simulink model "ModuladorTorqueEquivalente"  (R2023b)
settings: Solver=VariableStepAuto  StartTime=0.0  StopTime=10.0  RelTol=1e-3
values from neighbouring files (symbols this model uses):
  b_eq = b_m + b_l/(r^2)    (= 2.19444444444e-05)    [Parametros.m]
  k_l = m*l_cm + m_l(1)*l_l    [Parametros.m]
  L_d = 6.6E-3    (= 0.0066)    [Parametros.m]
  L_ls = 0.8E-3    (= 0.0008)    [Parametros.m]
  L_q = 5.8E-3    (= 0.0058)    [Parametros.m]
  lambda_m = 0.016    [Parametros.m]
  P_p = 3    [Parametros.m]
  r = 120    [MigracionPolosControladorExterno.m]    (also in Parametros.m)
settings Model: Creator=matia  LastModifiedBy=matia

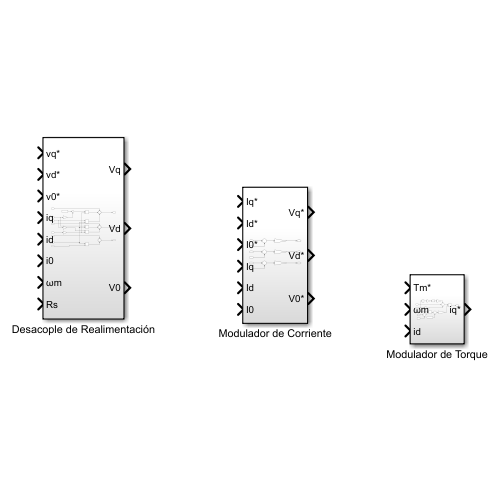
[thumbnail: Simulink's stored preview of the top-level diagram]
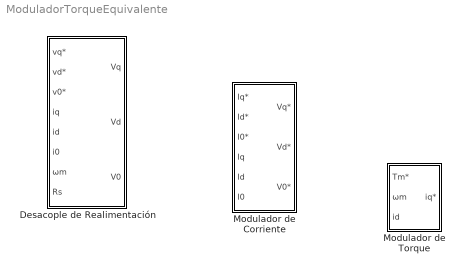
== system ModuladorTorqueEquivalente ==
  Desacople de Realimentación : Subsystem
  Modulador de Corriente : Subsystem
  Modulador de Torque : Subsystem

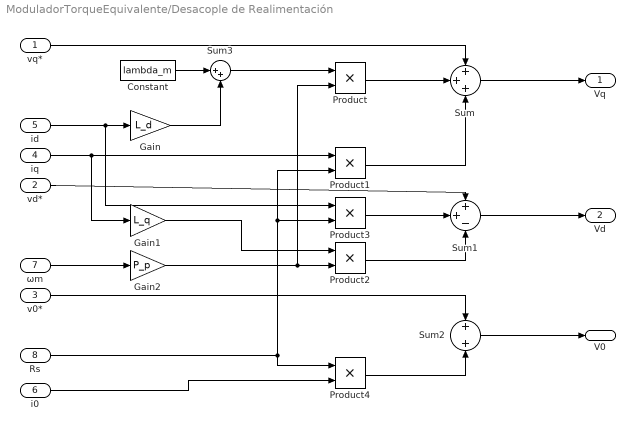
== system ModuladorTorqueEquivalente/Desacople de Realimentación ==
  vq* : Inport
  vd* : Inport  Port=2
  v0* : Inport  Port=3
  iq : Inport  Port=4
  id : Inport  Port=5
  i0 : Inport  Port=6
  ωm : Inport  Port=7
  Rs : Inport  Port=8
  Constant : Constant  Value=lambda_m
  Gain : Gain  Gain=L_d
  Gain1 : Gain  Gain=L_q
  Gain2 : Gain  Gain=P_p
  Product{,1..4} (5 alike) : Product
  Sum : Sum  Inputs=+++
  Sum1 : Sum  Inputs=++-
  Sum2 : Sum  Inputs=+|+
  Sum3 : Sum  Inputs=|++
  Vq : Outport
  Vd : Outport  Port=2
  V0 : Outport  Port=3
  wires:
  ωm/1 -> Gain2/1
  Sum/1 -> Vq/1
  Rs/1 -> Product4/1, Product1/2, Product3/2
  Gain/1 -> Sum3/2
  Product/1 -> Sum/2
  Sum2/1 -> V0/1
  Product4/1 -> Sum2/2
  Sum3/1 -> Product/1
  id/1 -> Product3/1, Gain/1
  vq*/1 -> Sum/1
  i0/1 -> Product4/2
  iq/1 -> Product1/1, Gain1/1
  Product2/1 -> Sum1/3
  Constant/1 -> Sum3/1
  v0*/1 -> Sum2/1
  Product1/1 -> Sum/3
  Gain2/1 -> Product/2, Product2/2
  vd*/1 -> Sum1/1
  Gain1/1 -> Product2/1
  Sum1/1 -> Vd/1
  Product3/1 -> Sum1/2

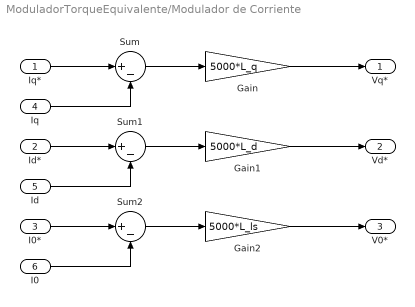
== system ModuladorTorqueEquivalente/Modulador de Corriente ==
  Iq* : Inport
  Id* : Inport  Port=2
  I0* : Inport  Port=3
  Iq : Inport  Port=4
  Id : Inport  Port=5
  I0 : Inport  Port=6
  Gain : Gain  Gain=5000*L_q
  Gain1 : Gain  Gain=5000*L_d
  Gain2 : Gain  Gain=5000*L_ls
  Sum : Sum  Inputs=|+-
  Sum1 : Sum  Inputs=|+-
  Sum2 : Sum  Inputs=|+-
  Vq* : Outport
  Vd* : Outport  Port=2
  V0* : Outport  Port=3
  wires:
  Gain2/1 -> V0*/1
  Sum/1 -> Gain/1
  Sum1/1 -> Gain1/1
  Gain/1 -> Vq*/1
  Iq/1 -> Sum/2
  I0*/1 -> Sum2/1
  Iq*/1 -> Sum/1
  Id/1 -> Sum1/2
  Sum2/1 -> Gain2/1
  Id*/1 -> Sum1/1
  Gain1/1 -> Vd*/1
  I0/1 -> Sum2/2

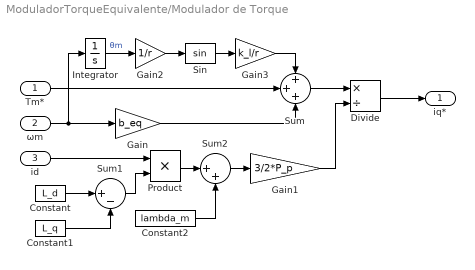
== system ModuladorTorqueEquivalente/Modulador de Torque ==
  Tm* : Inport
  ωm : Inport  Port=2
  id : Inport  Port=3
  Constant : Constant  Value=L_d
  Constant1 : Constant  Value=L_q
  Constant2 : Constant  Value=lambda_m
  Divide : Product  Inputs=*/
  Gain : Gain  Gain=b_eq
  Gain1 : Gain  Gain=3/2*P_p
  Gain2 : Gain  Gain=1/r
  Gain3 : Gain  Gain=k_l/r
  Integrator : Integrator
  Product : Product
  Sin : Trigonometry
  Sum : Sum  Inputs=+++
  Sum1 : Sum  Inputs=|+-
  Sum2 : Sum  Inputs=|++
  iq* : Outport
  wires:
  Constant2/1 -> Sum2/2
  ωm/1 -> Gain/1, Integrator/1
  Sum1/1 -> Product/2
  Gain3/1 -> Sum/1
  Integrator/1 -> Gain2/1  "θm"
  Sum2/1 -> Gain1/1
  Constant/1 -> Sum1/1
  Gain1/1 -> Divide/2
  Divide/1 -> iq*/1
  Product/1 -> Sum2/1
  Gain/1 -> Sum/3
  Constant1/1 -> Sum1/2
  Sin/1 -> Gain3/1
  Gain2/1 -> Sin/1
  Sum/1 -> Divide/1
  id/1 -> Product/1
  Tm*/1 -> Sum/2
